simulink subsystem "Subsystem_2S"  (R2025b)
settings: Solver=VariableStepAuto  StartTime=0.0  StopTime=10.0  RelTol=1e-3
model mask{station_order=0, RainSwitch_S1=on, flip_order=off, Waterlevel_1=275, Height=1, K=7.77*1e-5, Max_cap_1=300, Diameter=24.5, BurstStart=1, BurstFlow=1, BurstDur=1, rain_start=0, Duration_S1=10, Flowrate_S1=1, A=0.0117, B=0.1252, Parameter37=0, Parameter35=0, Parameter36=0, Parameter38=0, Parameter39=0, Waterlevel_2=150, Height_2=1, Max_cap_2=300, Diameter_2=24.5, K_2=7.77*1e-5, A_2=0.0117, B_2=0.1252, Duration_S2=10, Flowrate_S2=1, BurstStart_2=1, BurstFlow_2=1, BurstDur_2=1, rain_start_2=0, station_order_2=0, flip_order_2=off, RainSwitch_S2=on, DelayLength=0, EnableBurst=on}
  mask prompts: station_order "Station order:"; RainSwitch_S1 "Set rain on/off"; flip_order "Flip order"; Waterlevel_1 "Initial water level (mm):"; Height "Altitude (m):"; K "K Coefficient:"; Max_cap_1 "Height (mm):"; Diameter "Diameter (cm):"; BurstStart "Burst start (sec):"; BurstFlow "Burst flow (liters/min):"; BurstDur "Burst duration (sec):"; rain_start "Rain start (sec):"; Duration_S1 "Rain duration (sec):"; Flowrate_S1 "Rain flowrate (liters/min):"; A "G(u(t)) ="; B "u(t) -"; Waterlevel_2 "Initial water level:"; Height_2 "Height:"; Max_cap_2 "Max capacity:"; Diameter_2 "Diameter:"; K_2 "K:"; A_2 "Valve coeff A:"; B_2 "B:"; Duration_S2 "Duration (sec):"; Flowrate_S2 "Flowrate (liters/min):"; BurstStart_2 "Burst start:"; BurstFlow_2 "Burst flow:"; BurstDur_2 "Burst duration:"; rain_start_2 "Rain start (sec):"; station_order_2 "Station order:"; flip_order_2 "Flip order"; RainSwitch_S2 "Set rain on/off"; DelayLength "Transport delay(sec):"; EnableBurst "Enable cloud burst"
settings Model: Creator=klump  LastModifiedBy=klump

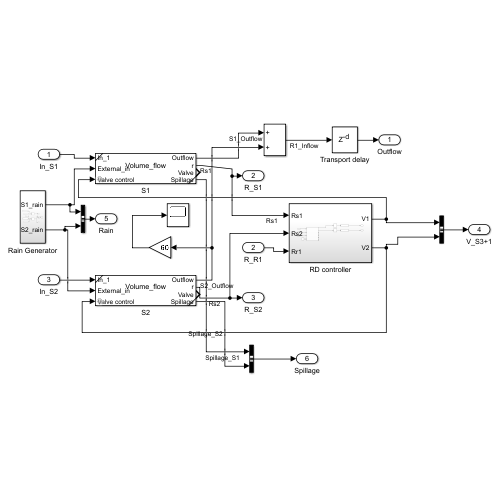
[thumbnail: Simulink's stored preview of the top-level diagram]
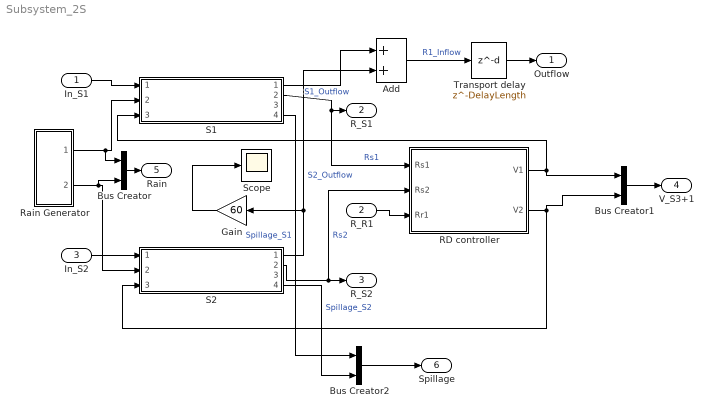
== system Subsystem_2S ==
  In_S1 : Inport
  R_R1 : Inport  Port=2
  In_S2 : Inport  Port=3
  Add : Sum
  Bus Creator : BusCreator  Inputs=2
  Bus Creator1 : BusCreator  Inputs=2
  Bus Creator2 : BusCreator  Inputs=2
  Gain : Gain  Gain=60
  RD controller : Subsystem
  Rain Generator : Subsystem
  S1 : Subsystem  ReferencedSubsystem=Volume_flow  InitialCondition=Waterlevel_1  Max_cap=Max_cap_1  Diameter=Diameter  K=K  Height=Height  A=A  B=B
  S2 : Subsystem  ReferencedSubsystem=Volume_flow  InitialCondition=Waterlevel_2  Max_cap=Max_cap_2  Diameter=Diameter_2  K=K_2  Height=Height_2  A=A_2  B=B_2
  Scope : Scope
      settings: ActiveDisplayYMinimum=-1  ActiveDisplayYMaximum=1  DataLoggingVariableName=ScopeData23
  Transport delay : Delay  DelayLength=DelayLength  InputProcessing=Columns as channels (frame based)
  Outflow : Outport
  R_S1 : Outport  Port=2
  R_S2 : Outport  Port=3
  V_S3+1 : Outport  Port=4
  Rain : Outport  Port=5
  Spillage : Outport  Port=6
  wires:
  In_S2/1 -> S2/1
  R_R1/1 -> RD controller/3(Rr1)
  S2/2 -> R_S2/1, RD controller/2(Rs2)  "Rs2"
  Bus Creator1/1 -> V_S3+1/1
  Add/1 -> Transport delay/1  "R1_Inflow"
  Transport delay/1 -> Outflow/1
  S2/1 -> Add/2, Gain/1  "S2_Outflow"
  S1/2 -> R_S1/1, RD controller/1(Rs1)  "Rs1"
  S1/1 -> Add/1  "S1_Outflow"
  RD controller/1(V1) -> S1/3, Bus Creator1/1
  Rain Generator/1(S1_rain) -> S1/2, Bus Creator/1
  In_S1/1 -> S1/1
  Rain Generator/2(S2_rain) -> S2/2, Bus Creator/2
  RD controller/2(V2) -> Bus Creator1/2, S2/3
  Gain/1 -> Scope/1
  Bus Creator/1 -> Rain/1
  Bus Creator2/1 -> Spillage/1
  S2/4 -> Bus Creator2/2  "Spillage_S2"
  S1/4 -> Bus Creator2/1  "Spillage_S1"

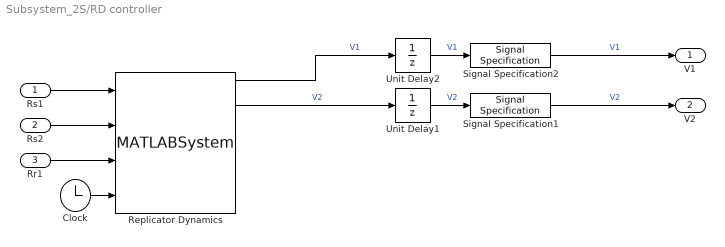
== system Subsystem_2S/RD controller ==
  Rs1 : Inport
  Rs2 : Inport  Port=2
  Rr1 : Inport  Port=3
  Clock : Clock
  Replicator Dynamics : MATLABSystem  System=RD_controller  SimulateUsing=Interpreted execution
      mask Type: RD_controller
  Signal Specification1 : SignalSpecification  Dimensions=1
  Signal Specification2 : SignalSpecification  Dimensions=1
  Unit Delay1 : UnitDelay  SampleTime=-1  HasFrameUpgradeWarning=on
  Unit Delay2 : UnitDelay  SampleTime=-1  HasFrameUpgradeWarning=on
  V1 : Outport
  V2 : Outport  Port=2
  wires:
  Rr1/1 -> Replicator Dynamics/3
  Rs2/1 -> Replicator Dynamics/2
  Rs1/1 -> Replicator Dynamics/1
  Clock/1 -> Replicator Dynamics/4
  Unit Delay2/1 -> Signal Specification2/1  "V1"
  Signal Specification2/1 -> V1/1  "V1"
  Unit Delay1/1 -> Signal Specification1/1  "V2"
  Signal Specification1/1 -> V2/1  "V2"
  Replicator Dynamics/2 -> Unit Delay1/1  "V2"
  Replicator Dynamics/1 -> Unit Delay2/1  "V1"

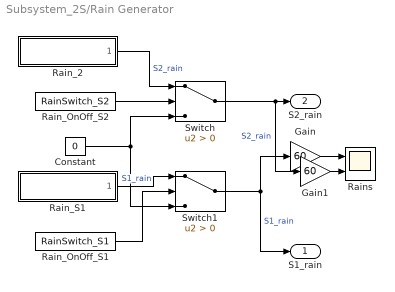
== system Subsystem_2S/Rain Generator ==
  Constant : Constant  Value=0
  Gain : Gain  Gain=60
  Gain1 : Gain  Gain=60
  Rain_2 : Subsystem  ReferencedSubsystem=Rain  Duration=Duration_S2  Flowrate=Flowrate_S2  BurstStart=BurstStart_2  BurstFlow=BurstFlow_2  BurstDur=BurstDur_2  flip_order=off  rain_start=rain_start_2  station_order=station_order_2  EnableBurst=on
  Rain_OnOff_S1 : Constant  Value=RainSwitch_S1
  Rain_OnOff_S2 : Constant  Value=RainSwitch_S2
  Rain_S1 : Subsystem  ReferencedSubsystem=Rain  Duration=Duration_S1  Flowrate=Flowrate_S1  BurstStart=BurstStart  BurstFlow=BurstFlow  BurstDur=BurstDur  flip_order=off  rain_start=rain_start  station_order=station_order  EnableBurst=on
  Rains : Scope  NumInputPorts=2
      settings: ActiveDisplayYMinimum=-0.5  ActiveDisplayYMaximum=20.5  YLabel=Flowrate (liters/minute)  DataLoggingVariableName=ScopeData2
  Switch : Switch  Criteria=u2 > Threshold  SaturateOnIntegerOverflow=off  InputSameDT=off
  Switch1 : Switch  Criteria=u2 > Threshold  SaturateOnIntegerOverflow=off  InputSameDT=off
  S1_rain : Outport
  S2_rain : Outport  Port=2
  wires:
  Gain1/1 -> Rains/2
  Gain/1 -> Rains/1
  Rain_OnOff_S1/1 -> Switch1/2
  Rain_2/1 -> Switch/1  "S2_rain"
  Rain_S1/1 -> Switch1/1  "S1_rain"
  Constant/1 -> Switch1/3, Switch/3
  Switch1/1 -> S1_rain/1, Gain/1  "S1_rain"
  Rain_OnOff_S2/1 -> Switch/2
  Switch/1 -> S2_rain/1, Gain1/1  "S2_rain"
